simulink model "sampleModel147"  (R2021b)
settings: Solver=VariableStepAuto  StartTime=0.0  StopTime=10.0  RelTol=1e-3
undefined symbols (not defined in the file or in its folder): Newton, Raphson
libraries: simulink x2
settings Model: Creator=user  LastModifiedBy=user

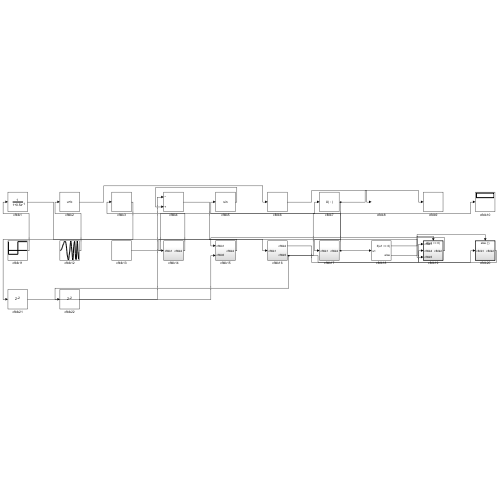
[thumbnail: Simulink's stored preview of the top-level diagram]
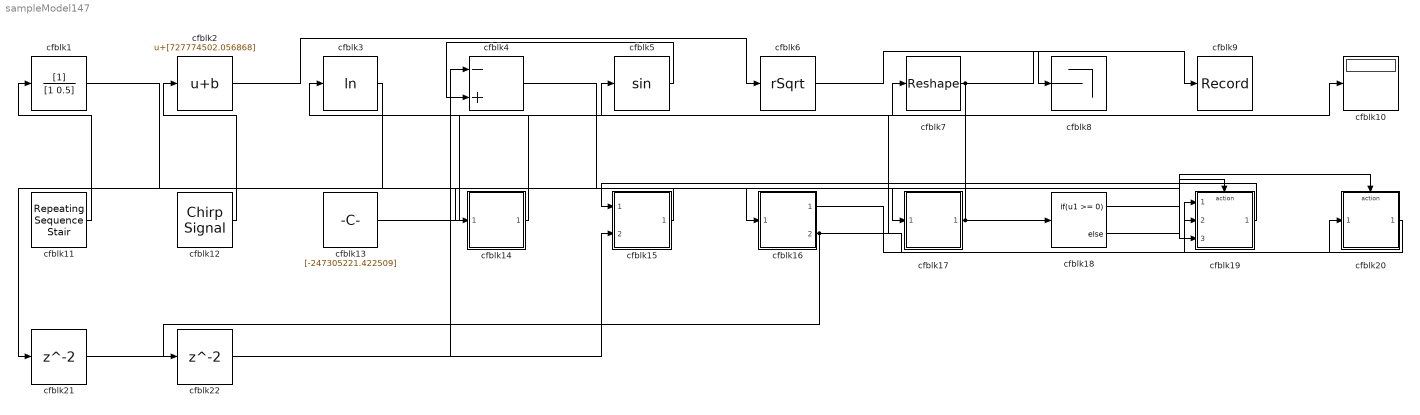
== system sampleModel147 ==
  cfblk1 : DiscreteFilter  SampleTime=1
  cfblk10 : Display
  cfblk11 : simulink/Sources/Repeating Sequence Stair  OutValues=[-397227382.137541, 938260549.234686]  tsamp=-1  OutMin=[]  OutMax=[]  OutDataTypeStr=double  OutputDataTypeScalingMode=double  OutDataType=fixdt(0,8)  ConRadixGroup=Best Precision: Vector-wise  OutScaling=2^-12
  cfblk12 : simulink/Sources/Chirp Signal  f1=[685992920.395310]  T=[-837548117.846636]  f2=[169290031.686611]
  cfblk13 : Constant  Value=[-247305221.422509]  SampleTime=1
  cfblk14 : Subsystem
  cfblk15 : Subsystem
  cfblk16 : Subsystem
  cfblk17 : Subsystem
  cfblk18 : If  IfExpression=u1 >= 0  SampleTime=1
  cfblk19 : Subsystem  TreatAsAtomicUnit=on
  cfblk2 : Bias  Bias=[727774502.056868]
  cfblk20 : Subsystem  TreatAsAtomicUnit=on
  cfblk21 : Delay  SampleTime=1
  cfblk22 : Delay  SampleTime=1
  cfblk3 : Math  Operator=log  SaturateOnIntegerOverflow=on
  cfblk4 : Sum  Inputs=-+
  cfblk5 : Trigonometry
  cfblk6 : Sqrt  Operator=rSqrt  AlgorithmType=Newton-Raphson  SaturateOnIntegerOverflow=on
  cfblk7 : Reshape
  cfblk8 : Terminator
  cfblk9 : Record  FileSettingsInternal="{\"entries\":[{\"content\":{\"excelSettings\":{\"content\":{},\"type\":\"Streamout.ExcelSettings\"}},\"type\":\"Streamout.FileSettingStorage\",\"uuid\":\"e5de7313-9b70-49f3-b795-696202b7e5ee\"}],\"packageUris\":[\"http://schema.mathworks.com/mf0/streamout_blocks/R2020a\"],\"version\":\"1.0\"}"  SignalsInternal="{\"entries\":[{\"content\":{\"signals\":[{\"content\":{\"blockPath\":[\"sampleModel147/cfblk9\"],\"channel\":[],\"dimensions\":[1],\"domain\":\"sampleModel147/cfblk9\",\"lineColor\":\"#0072bd\",\"plots\":[1],\"port\":1,\"sid\":[\"\"],\"signalID\":5320,\"signalName\":\"cfblk7\"},\"type\":\"RecordBlkView.Signal\",\"uuid\":\"355f090d-3d63-44f9-9a60-b05337dbe9e4\"}]},\"type\":\"RecordBlkView.InputSignals\",\"uuid\":\"92d60f7a-f4b0-42b1-b8d3-4c4b9f409310\"}],\"packageUris\":[\"http://schema.mathworks.com/mf0/streamout_blocks/R2020a\"],\"version\":\"1.0\"}"  VisualizationBindings="{\"sparklinesplugin\":{\"info\":[{\"bindingParametersList\":[],\"subplotID\":1}]}}"
  wires:
  cfblk19/1(cfblk2) -> cfblk15/1(cfblk1)
  cfblk7/1 -> cfblk17/1(cfblk1), cfblk9/1
  cfblk14/1(cfblk2) -> cfblk3/1
  cfblk16/1(cfblk2) -> cfblk19/1(cfblk1)
  cfblk20/1(cfblk2) -> cfblk19/2(cfblk4)
  cfblk17/1(cfblk2) -> cfblk5/1, cfblk18/1
  cfblk16/2(cfblk5) -> cfblk20/1(cfblk1), cfblk10/1, cfblk22/1
  cfblk13/1 -> cfblk7/1
  cfblk12/1 -> cfblk2/1
  cfblk6/1 -> cfblk8/1
  cfblk15/1(cfblk2) -> cfblk14/1(cfblk1)
  cfblk1/1 -> cfblk19/3(cfblk5)
  cfblk4/1 -> cfblk16/1(cfblk1)
  cfblk5/1 -> cfblk4/2
  cfblk11/1 -> cfblk1/1
  cfblk2/1 -> cfblk6/1
  cfblk18/1 -> cfblk19/Action
  cfblk18/2 -> cfblk20/Action
  cfblk3/1 -> cfblk21/1
  cfblk21/1 -> cfblk15/2(cfblk5)
  cfblk22/1 -> cfblk4/1

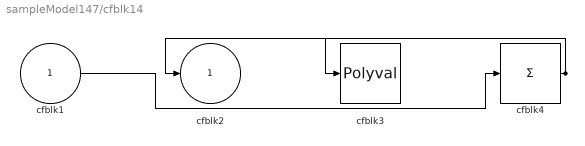
== system sampleModel147/cfblk14 ==
  cfblk1 : Inport
  cfblk3 : Polyval  Coefs=[ +2.081618890e-019, -1.441693666e-014, +4.719686976e-010, -8.536869453e-006, +1.621573104e-001, -8.087801117e+001 ]
  cfblk4 : Sum  Inputs=+
  cfblk2 : Outport
  wires:
  cfblk4/1 -> cfblk2/1, cfblk3/1
  cfblk1/1 -> cfblk4/1

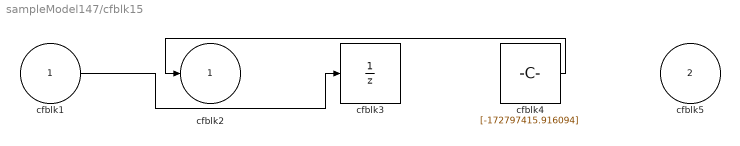
== system sampleModel147/cfblk15 ==
  cfblk1 : Inport
  cfblk5 : Inport  Port=2
  cfblk3 : UnitDelay  HasFrameUpgradeWarning=on
  cfblk4 : Constant  Value=[-172797415.916094]  SampleTime=1
  cfblk2 : Outport
  wires:
  cfblk4/1 -> cfblk2/1
  cfblk1/1 -> cfblk3/1

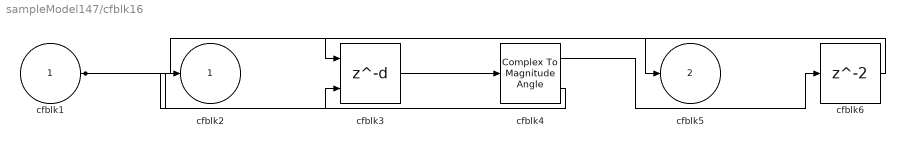
== system sampleModel147/cfblk16 ==
  cfblk1 : Inport
  cfblk3 : Delay  DelayLengthSource=Input port  SampleTime=1
      settings: InputPortMap=u0,p1
  cfblk4 : ComplexToMagnitudeAngle
  cfblk6 : Delay  SampleTime=1
  cfblk2 : Outport
  cfblk5 : Outport  Port=2
  wires:
  cfblk1/1 -> cfblk5/1, cfblk3/2
  cfblk4/2 -> cfblk2/1
  cfblk3/1 -> cfblk4/1
  cfblk4/1 -> cfblk6/1
  cfblk6/1 -> cfblk3/1

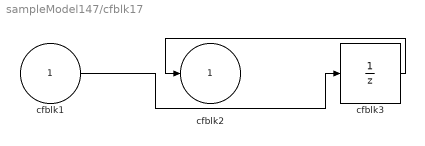
== system sampleModel147/cfblk17 ==
  cfblk1 : Inport
  cfblk3 : UnitDelay  HasFrameUpgradeWarning=on
  cfblk2 : Outport
  wires:
  cfblk3/1 -> cfblk2/1
  cfblk1/1 -> cfblk3/1

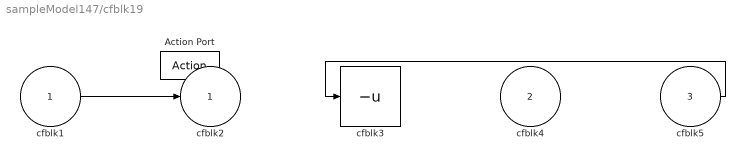
== system sampleModel147/cfblk19 ==
  cfblk1 : Inport
  cfblk4 : Inport  Port=2
  cfblk5 : Inport  Port=3
  Action Port : ActionPort  ActionPortLabel=if(u1 >= 0)
  cfblk3 : UnaryMinus
  cfblk2 : Outport
  wires:
  cfblk1/1 -> cfblk2/1
  cfblk5/1 -> cfblk3/1

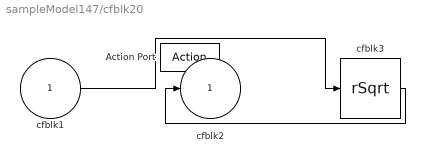
== system sampleModel147/cfblk20 ==
  cfblk1 : Inport
  Action Port : ActionPort  ActionPortLabel=else
  cfblk3 : Sqrt  Operator=rSqrt  AlgorithmType=Newton-Raphson  SaturateOnIntegerOverflow=on
  cfblk2 : Outport
  wires:
  cfblk3/1 -> cfblk2/1
  cfblk1/1 -> cfblk3/1
